simulink model "audio_band_adc"  (R2021a)
settings: Solver=FixedStepAuto  StartTime=0.0  StopTime=10.0  RelTol=1e-3
undefined symbols (not defined in the file): Fs, modctrl
libraries: dspsrcs4 x4
settings Model: Creator=samir  LastModifiedBy=samir
settings ModelReferenceCC: ModelReferenceNumInstancesAllowed=Single

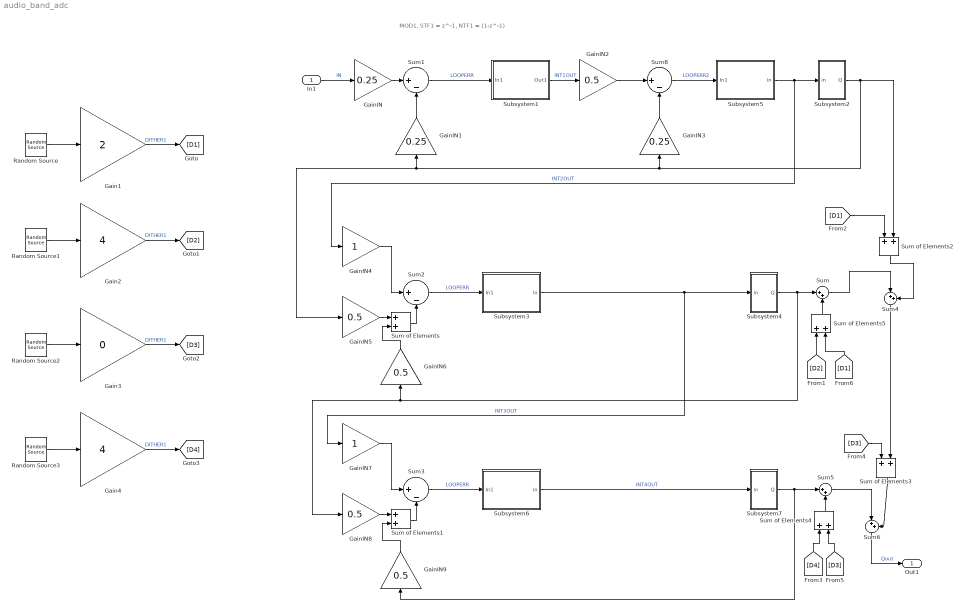
== system audio_band_adc ==
  note: MOD1, STF1 = z^-1, NTF1 = (1-z^-1)
  In1 : Inport
  Gain1 : Gain  Gain=2
      settings: AttributesFormatString=Dither level adjust
  Gain2 : Gain  Gain=4
      settings: AttributesFormatString=Dither level adjust
  Gain3 : Gain  Gain=0
      settings: AttributesFormatString=Dither level adjust
  Gain4 : Gain  Gain=4
      settings: AttributesFormatString=Dither level adjust
  GainIN : Gain  Gain=0.25
  GainIN1 : Gain  Gain=0.25
  GainIN{2,5..6,8..9} (5 alike) : Gain  Gain=0.5
  GainIN3 : Gain  Gain=0.25
  GainIN4 : Gain
  GainIN7 : Gain
  Random Source{,1..3} (4 alike) : dspsrcs4/Random Source  SrcType=Uniform  NormMethod=Ziggurat  CltLength=12  MinVal=-1  MaxVal=1  MeanVal=0  VarVal=1  RepMode=Not repeatable  rawSeed=1  IsInherit=off  SampMode=Discrete  SampTime=1/Fs  SampFrame=1  DataType=Double  OutComplex=Real  OutputFrames=on
      settings: AttributesFormatString=Dither source
  Subsystem1 : Subsystem
      settings: AttributesFormatString=Leaky delaying int
  Subsystem2 : Subsystem
      settings: AttributesFormatString=2-bit quantiser
  Subsystem3 : Subsystem
      settings: AttributesFormatString=Leaky delaying int
  Subsystem4 : Subsystem
      settings: AttributesFormatString=2-bit quantiser
  Subsystem5 : Subsystem
      settings: AttributesFormatString=Leaky delaying int
  Subsystem6 : Subsystem
      settings: AttributesFormatString=Leaky delaying int
  Subsystem7 : Subsystem
      settings: AttributesFormatString=2-bit quantiser
  Sum{,4..6} (4 alike) : Sum  Inputs=|++
  Sum of Elements{,1..5} (6 alike) : Sum
  Sum{1..3,8} (4 alike) : Sum  Inputs=|+-
      settings: AttributesFormatString=Modulator input\nloop servo error (input - fbk)
  Out1 : Outport  SignalName=Out
  wires:
  Sum1/1 -> Subsystem1/1(In1)  "LOOPERR"
  Sum8/1 -> Subsystem5/1(In1)  "LOOPERR2"
  In1/1 -> GainIN/1  "IN"
  GainIN/1 -> Sum1/1
  GainIN1/1 -> Sum1/2
  Subsystem1/1(Out1) -> GainIN2/1  "INT1OUT"
  GainIN2/1 -> Sum8/1
  GainIN3/1 -> Sum8/2
  Subsystem5/1(in) -> GainIN4/1, Subsystem2/1(in)  "INT2OUT"
  GainIN4/1 -> Sum2/1
  GainIN5/1 -> Sum of Elements/1
  Subsystem2/1(Q) -> Sum of Elements2/2, GainIN1/1, GainIN5/1, GainIN3/1
  Sum2/1 -> Subsystem3/1(In1)  "LOOPERR"
  Sum of Elements/1 -> Sum2/2
  GainIN6/1 -> Sum of Elements/2
  Subsystem3/1(in) -> GainIN7/1, Subsystem4/1(in)  "INT3OUT"
  GainIN9/1 -> Sum of Elements1/2
  GainIN7/1 -> Sum3/1
  Sum3/1 -> Subsystem6/1(In1)  "LOOPERR"
  GainIN8/1 -> Sum of Elements1/1
  Sum of Elements1/1 -> Sum3/2
  Subsystem6/1(in) -> Subsystem7/1(in)  "INT4OUT"
  Subsystem7/1(Q) -> Sum5/1, GainIN9/1
  Subsystem4/1(Q) -> Sum/1, GainIN6/1, GainIN8/1
  Random Source/1 -> Gain1/1
  Gain1/1 -> [D1]  "DITHER1"
  Gain2/1 -> [D2]  "DITHER1"
  Random Source1/1 -> Gain2/1
  Random Source2/1 -> Gain3/1
  Gain3/1 -> [D3]  "DITHER1"
  Random Source3/1 -> Gain4/1
  Gain4/1 -> [D4]  "DITHER1"
  Sum/1 -> Sum4/1
  [D1] -> Sum of Elements2/1
  Sum of Elements2/1 -> Sum4/2
  Sum5/1 -> Sum6/1
  Sum of Elements3/1 -> Sum6/2
  [D3] -> Sum of Elements3/1
  Sum4/1 -> Sum of Elements3/2
  Sum6/1 -> Out1/1  "Qout"
  [D4] -> Sum of Elements4/1
  [D3] -> Sum of Elements4/2
  Sum of Elements4/1 -> Sum5/2
  [D2] -> Sum of Elements5/1
  [D1] -> Sum of Elements5/2
  Sum of Elements5/1 -> Sum/2

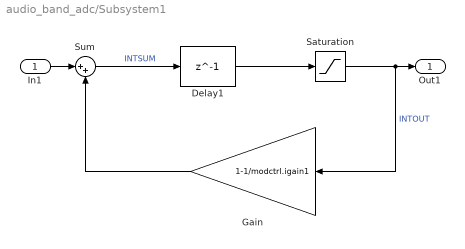
== system audio_band_adc/Subsystem1 ==
  In1 : Inport
  Delay1 : Delay  DelayLength=1  InitialCondition=0
  Gain : Gain  Gain=1-1/modctrl.igain1
      settings: AttributesFormatString=Integrator leakage
  Saturation : Saturate  UpperLimit=modctrl.isat1  LowerLimit=-(modctrl.isat1)
  Sum : Sum  Inputs=|++
      settings: AttributesFormatString=Integrator summer
  Out1 : Outport
  wires:
  Sum/1 -> Delay1/1  "INTSUM"
  Gain/1 -> Sum/2
  Saturation/1 -> Gain/1, Out1/1  "INTOUT"
  Delay1/1 -> Saturation/1
  In1/1 -> Sum/1

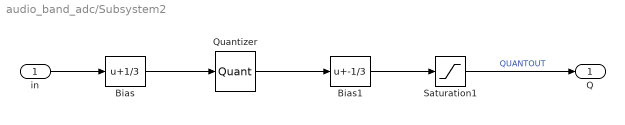
== system audio_band_adc/Subsystem2 ==
  in : Inport
  Bias : Bias  Bias=1/3
      settings: AttributesFormatString=Need offset to give\nMID-RISE quantiser
  Bias1 : Bias  Bias=-1/3
  Quantizer : Quantizer  QuantizationInterval=2/3  LinearizeAsGain=off
  Saturation1 : Saturate  UpperLimit=1  LowerLimit=-1
      settings: AttributesFormatString=Limit quantiser\noutput to +/-1
  Q : Outport
  wires:
  Bias/1 -> Quantizer/1
  Quantizer/1 -> Bias1/1
  Bias1/1 -> Saturation1/1
  in/1 -> Bias/1
  Saturation1/1 -> Q/1  "QUANTOUT"

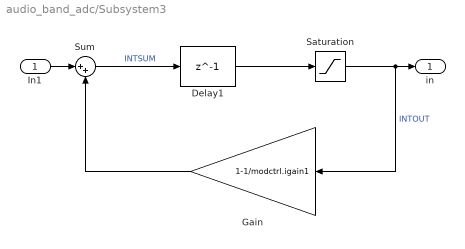
== system audio_band_adc/Subsystem3 ==
  In1 : Inport
  Delay1 : Delay  DelayLength=1  InitialCondition=0
  Gain : Gain  Gain=1-1/modctrl.igain1
      settings: AttributesFormatString=Integrator leakage
  Saturation : Saturate  UpperLimit=modctrl.isat1  LowerLimit=-(modctrl.isat1)
  Sum : Sum  Inputs=|++
      settings: AttributesFormatString=Integrator summer
  in : Outport
  wires:
  Sum/1 -> Delay1/1  "INTSUM"
  Gain/1 -> Sum/2
  Saturation/1 -> Gain/1, in/1  "INTOUT"
  Delay1/1 -> Saturation/1
  In1/1 -> Sum/1

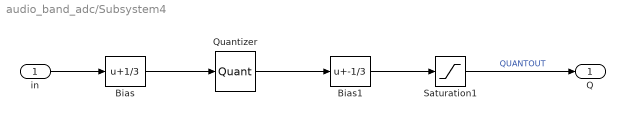
== system audio_band_adc/Subsystem4 ==
  in : Inport
  Bias : Bias  Bias=1/3
      settings: AttributesFormatString=Need offset to give\nMID-RISE quantiser
  Bias1 : Bias  Bias=-1/3
  Quantizer : Quantizer  QuantizationInterval=2/3  LinearizeAsGain=off
  Saturation1 : Saturate  UpperLimit=1  LowerLimit=-1
      settings: AttributesFormatString=Limit quantiser\noutput to +/-1
  Q : Outport
  wires:
  Bias/1 -> Quantizer/1
  Quantizer/1 -> Bias1/1
  Bias1/1 -> Saturation1/1
  in/1 -> Bias/1
  Saturation1/1 -> Q/1  "QUANTOUT"

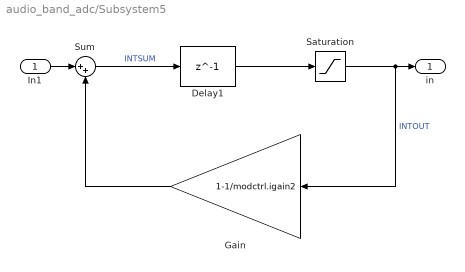
== system audio_band_adc/Subsystem5 ==
  In1 : Inport
  Delay1 : Delay  DelayLength=1  InitialCondition=0
  Gain : Gain  Gain=1-1/modctrl.igain2
      settings: AttributesFormatString=Integrator leakage
  Saturation : Saturate  UpperLimit=modctrl.isat2  LowerLimit=-(modctrl.isat2)
  Sum : Sum  Inputs=|++
      settings: AttributesFormatString=Integrator summer
  in : Outport
  wires:
  In1/1 -> Sum/1
  Delay1/1 -> Saturation/1
  Saturation/1 -> in/1, Gain/1  "INTOUT"
  Gain/1 -> Sum/2
  Sum/1 -> Delay1/1  "INTSUM"

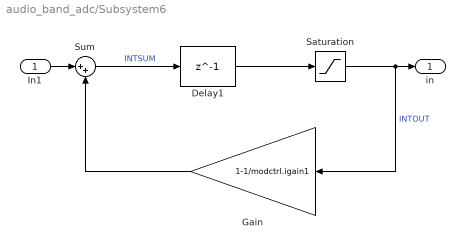
== system audio_band_adc/Subsystem6 ==
  In1 : Inport
  Delay1 : Delay  DelayLength=1  InitialCondition=0
  Gain : Gain  Gain=1-1/modctrl.igain1
      settings: AttributesFormatString=Integrator leakage
  Saturation : Saturate  UpperLimit=modctrl.isat1  LowerLimit=-(modctrl.isat1)
  Sum : Sum  Inputs=|++
      settings: AttributesFormatString=Integrator summer
  in : Outport
  wires:
  Sum/1 -> Delay1/1  "INTSUM"
  Gain/1 -> Sum/2
  Saturation/1 -> Gain/1, in/1  "INTOUT"
  Delay1/1 -> Saturation/1
  In1/1 -> Sum/1

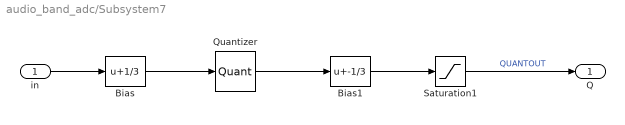
== system audio_band_adc/Subsystem7 ==
  in : Inport
  Bias : Bias  Bias=1/3
      settings: AttributesFormatString=Need offset to give\nMID-RISE quantiser
  Bias1 : Bias  Bias=-1/3
  Quantizer : Quantizer  QuantizationInterval=2/3  LinearizeAsGain=off
  Saturation1 : Saturate  UpperLimit=1  LowerLimit=-1
      settings: AttributesFormatString=Limit quantiser\noutput to +/-1
  Q : Outport
  wires:
  Bias/1 -> Quantizer/1
  Quantizer/1 -> Bias1/1
  Bias1/1 -> Saturation1/1
  in/1 -> Bias/1
  Saturation1/1 -> Q/1  "QUANTOUT"
